simulink model "quadrotor_dust"  (R2026a)
settings: Solver=ode4  StopTime=quad_stop_time  FixedStep=0.02
model workspace (MAT data in the model file):
  quad_model_id_default = 2
undefined symbols (not defined in the file): quad_model_id, quad_param_vec, quad_scenario_id, quad_x0
Description:
  | 粉尘浓度扰动四旋翼模型：通过 eta_T 和 eta_Q 折减旋翼推力及反扭矩效率，体现粉尘对动力输出的影响。
settings Model: Creator=audib  LastModifiedBy=audib

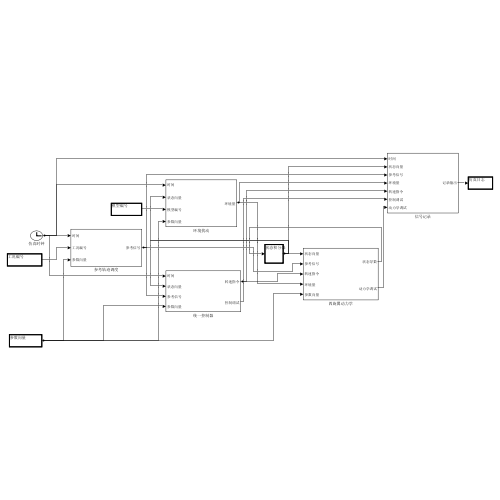
[thumbnail: Simulink's stored preview of the top-level diagram]
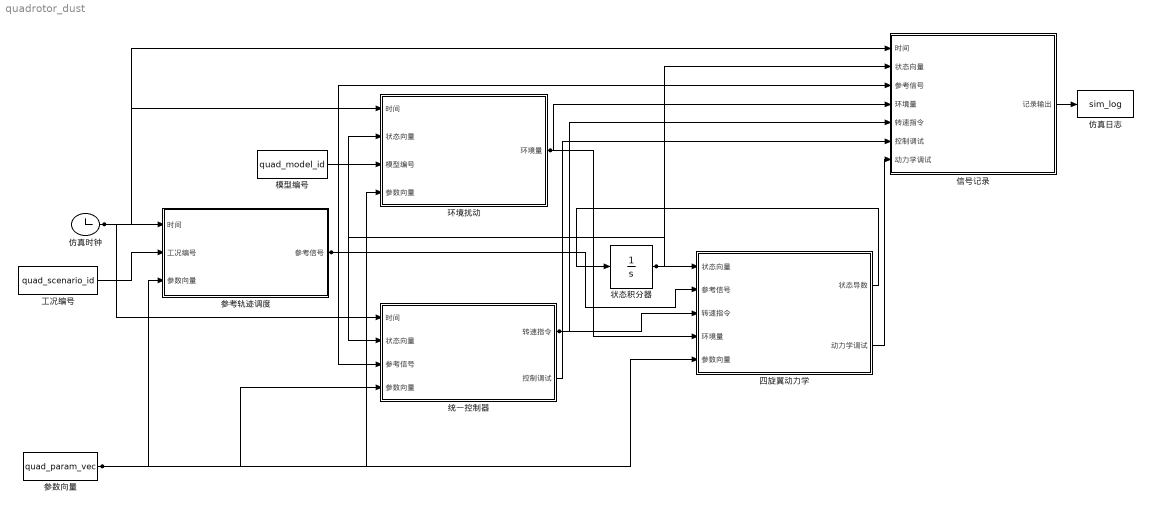
== system quadrotor_dust ==
  仿真日志 : ToWorkspace  VariableName=sim_log  SampleTime=-1
  仿真时钟 : Clock
  信号记录 : Subsystem
  参数向量 : Constant  Value=quad_param_vec
  参考轨迹调度 : Subsystem
  四旋翼动力学 : Subsystem
  工况编号 : Constant  Value=quad_scenario_id
  模型编号 : Constant  Value=quad_model_id
  状态积分器 : Integrator  InitialCondition=quad_x0
  环境扰动 : Subsystem
  统一控制器 : Subsystem
  wires:
  仿真时钟/1 -> 统一控制器/1(时间), 信号记录/1(时间), 环境扰动/1(时间), 参考轨迹调度/1(时间)
  模型编号/1 -> 环境扰动/3(模型编号)
  工况编号/1 -> 参考轨迹调度/2(工况编号)
  参考轨迹调度/1(参考信号) -> 信号记录/3(参考信号), 四旋翼动力学/2(参考信号), 统一控制器/3(参考信号)
  参数向量/1 -> 四旋翼动力学/5(参数向量), 参考轨迹调度/3(参数向量), 统一控制器/4(参数向量), 环境扰动/4(参数向量)
  环境扰动/1(环境量) -> 四旋翼动力学/4(环境量), 信号记录/4(环境量)
  统一控制器/2(控制调试) -> 信号记录/6(控制调试)
  统一控制器/1(转速指令) -> 四旋翼动力学/3(转速指令), 信号记录/5(转速指令)
  状态积分器/1 -> 环境扰动/2(状态向量), 统一控制器/2(状态向量), 信号记录/2(状态向量), 四旋翼动力学/1(状态向量)
  四旋翼动力学/1(状态导数) -> 状态积分器/1
  四旋翼动力学/2(动力学调试) -> 信号记录/7(动力学调试)
  信号记录/1(记录输出) -> 仿真日志/1

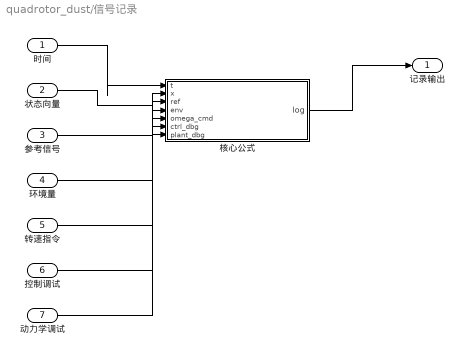
== system quadrotor_dust/信号记录 ==
  时间 : Inport
  状态向量 : Inport  Port=2
  参考信号 : Inport  Port=3
  环境量 : Inport  Port=4
  转速指令 : Inport  Port=5
  控制调试 : Inport  Port=6
  动力学调试 : Inport  Port=7
  核心公式 : MATLAB Function  TreatAsAtomicUnit=on
  记录输出 : Outport
  wires:
  时间/1 -> 核心公式/1(t)
  状态向量/1 -> 核心公式/2(x)
  参考信号/1 -> 核心公式/3(ref)
  环境量/1 -> 核心公式/4(env)
  转速指令/1 -> 核心公式/5(omega_cmd)
  控制调试/1 -> 核心公式/6(ctrl_dbg)
  动力学调试/1 -> 核心公式/7(plant_dbg)
  核心公式/1(log) -> 记录输出/1

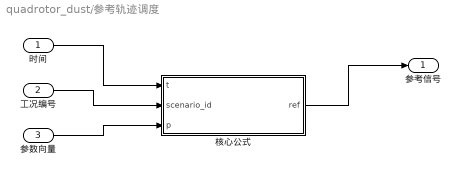
== system quadrotor_dust/参考轨迹调度 ==
  时间 : Inport
  工况编号 : Inport  Port=2
  参数向量 : Inport  Port=3
  核心公式 : MATLAB Function  TreatAsAtomicUnit=on
  参考信号 : Outport
  wires:
  时间/1 -> 核心公式/1(t)
  工况编号/1 -> 核心公式/2(scenario_id)
  参数向量/1 -> 核心公式/3(p)
  核心公式/1(ref) -> 参考信号/1

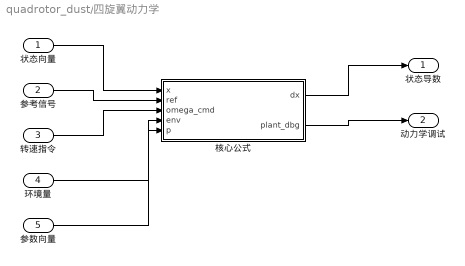
== system quadrotor_dust/四旋翼动力学 ==
  状态向量 : Inport
  参考信号 : Inport  Port=2
  转速指令 : Inport  Port=3
  环境量 : Inport  Port=4
  参数向量 : Inport  Port=5
  核心公式 : MATLAB Function  TreatAsAtomicUnit=on
  状态导数 : Outport
  动力学调试 : Outport  Port=2
  wires:
  状态向量/1 -> 核心公式/1(x)
  参考信号/1 -> 核心公式/2(ref)
  转速指令/1 -> 核心公式/3(omega_cmd)
  环境量/1 -> 核心公式/4(env)
  参数向量/1 -> 核心公式/5(p)
  核心公式/1(dx) -> 状态导数/1
  核心公式/2(plant_dbg) -> 动力学调试/1

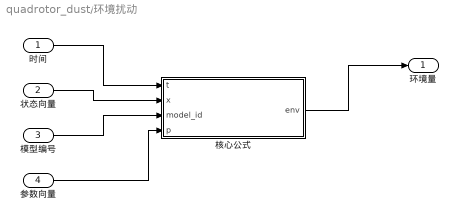
== system quadrotor_dust/环境扰动 ==
  时间 : Inport
  状态向量 : Inport  Port=2
  模型编号 : Inport  Port=3
  参数向量 : Inport  Port=4
  核心公式 : MATLAB Function  TreatAsAtomicUnit=on
  环境量 : Outport
  wires:
  时间/1 -> 核心公式/1(t)
  状态向量/1 -> 核心公式/2(x)
  模型编号/1 -> 核心公式/3(model_id)
  参数向量/1 -> 核心公式/4(p)
  核心公式/1(env) -> 环境量/1

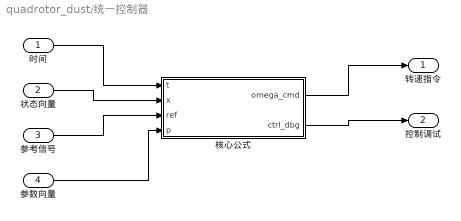
== system quadrotor_dust/统一控制器 ==
  时间 : Inport
  状态向量 : Inport  Port=2
  参考信号 : Inport  Port=3
  参数向量 : Inport  Port=4
  核心公式 : MATLAB Function  TreatAsAtomicUnit=on
  转速指令 : Outport
  控制调试 : Outport  Port=2
  wires:
  时间/1 -> 核心公式/1(t)
  状态向量/1 -> 核心公式/2(x)
  参考信号/1 -> 核心公式/3(ref)
  参数向量/1 -> 核心公式/4(p)
  核心公式/1(omega_cmd) -> 转速指令/1
  核心公式/2(ctrl_dbg) -> 控制调试/1

== matlab function quadrotor_dust/环境扰动/核心公式 ==
  data: t input; env output; x input; model_id input; p input
function env = fcn(t, x, model_id, p)
%#codegen
env = quadrotor_environment_core(t, x, model_id, p);
end

== matlab function quadrotor_dust/参考轨迹调度/核心公式 ==
  data: t input; ref output; scenario_id input; p input
function ref = fcn(t, scenario_id, p)
%#codegen
ref = quadrotor_reference_core(t, scenario_id, p);
end

== matlab function quadrotor_dust/统一控制器/核心公式 ==
  data: t input; omega_cmd output; x input; ref input; p input; ctrl_dbg output
function [omega_cmd, ctrl_dbg] = fcn(t, x, ref, p)
%#codegen
[omega_cmd, ctrl_dbg] = quadrotor_controller_core(t, x, ref, p);
end

== matlab function quadrotor_dust/四旋翼动力学/核心公式 ==
  data: x input; dx output; ref input; omega_cmd input; env input; p input; plant_dbg output
function [dx, plant_dbg] = fcn(x, ref, omega_cmd, env, p)
%#codegen
[dx, plant_dbg] = quadrotor_rhs_core(x, ref, omega_cmd, env, p);
end

== matlab function quadrotor_dust/信号记录/核心公式 ==
  data: t input; log output; x input; ref input; env input; omega_cmd input; ctrl_dbg input; plant_dbg input
function log = fcn(t, x, ref, env, omega_cmd, ctrl_dbg, plant_dbg)
%#codegen
log = quadrotor_pack_log_core(t, x, ref, env, omega_cmd, ctrl_dbg, plant_dbg);
end
